simulink model "PMSM_Sensorless_ASMO_PLL"  (R2024b)
settings: Solver=FixedStepAuto  StartTime=0.0  StopTime=0.2  FixedStep=1e-6  RelTol=1e-3
model workspace (MAT data in the model file):
  B = 0
  Current_Filter_On = 0
  F = 10000
  J = 5.8e-05
  Ls = 0.0005125
  PLL_Ki = 800
  PLL_Kp = 1000
  Pn = 5
  Rs = 0.1445
  T_deadband = 0
  Ts = 5e-05
  Vdc = 60
  id_ki = 5
  id_kp = 2.5
  iq_ki = 5
  iq_kp = 2.5
  k = 150
  l_asmo = 2000
  psi_f = 0.0113
  speed_ki = 5
  speed_kp = 0.2
  w_c = 8000
undefined symbols (not defined in the file): sigbuilder_block
libraries: dspfdesign x3, slpidlib x3, simulink x2, spsDCVoltageSourceLib x1, spsOnDelayLib x1, spsGroundLib x1, dsparch4 x1, spsPermanentMagnetSynchronousMachineLib x1, spsThreePhaseVIMeasurementLib x1, spsTwoLevelConverterLib x1, spspowerguiLib x1
settings Model: Creator=A  LastModifiedBy=31904
settings OptimizationCC: ReuseModelBlockBuffer=off
settings ModelReferenceCC: EnableRefExpFcnMdlSchedulingChecks=on
settings RTWCC: GPUComputeCapability=3.5

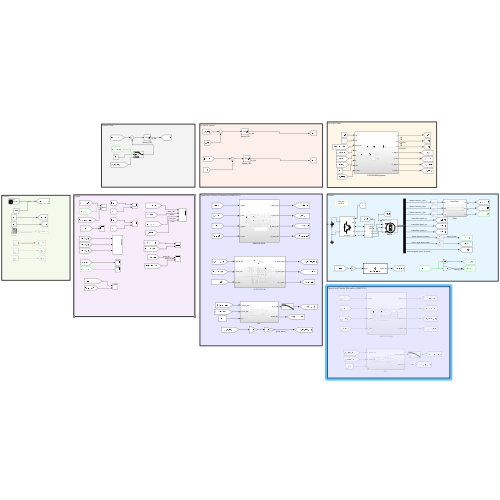
[thumbnail: Simulink's stored preview of the top-level diagram]
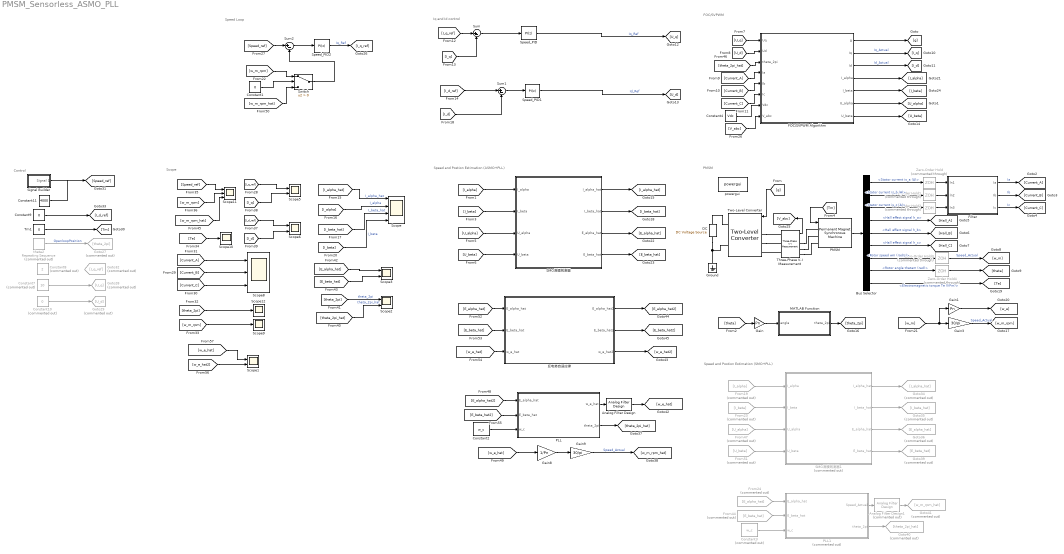
== system PMSM_Sensorless_ASMO_PLL ==
  note: Speed and Postion Estimation (ASMO+PLL)
  note: Iq and Id control
  note: FOC/SVPWM
  note: PMSM
  note: Speed Loop
  note: Control
  note: Scope
  note: Speed and Postion Estimation (SMO+PLL)
  Analog Filter Design : dspfdesign/Analog Filter Design  method=Butterworth  filttype=Lowpass  N=1  Wlo=8000  Whi=80  Rp=2  Rs=40
  Analog Filter Design1 : dspfdesign/Analog Filter Design  Commented=on  method=Butterworth  filttype=Lowpass  N=1  Wlo=8000  Whi=80  Rp=2  Rs=40
  Bus Selector : BusSelector  OutputSignals=Stator current is_a (A),Stator current is_b (A),Stator current is_c (A),Hall effect signal h_a,Hall effect signal h_b,Hall effect signal h_c,Rotor speed wm (rad/s),Rotor angle thetam (rad),Electromagnetic torque Te (N*m)
  Constant1 : Constant  Value=0
  Constant10 : Constant  Commented=on  Value=0
  Constant11 : Constant  Value=4000
  Constant2 : Constant  Value=w_c
  Constant3 : Constant  Commented=on  Value=w_c
  Constant4 : Constant  Value=Vdc
  Constant7 : Constant  Commented=on  Value=10
  Constant8 : Constant  Commented=on  Value=2
  Constant9 : Constant  Value=0
  DC : spsDCVoltageSourceLib/DC Voltage Source  Amplitude=Vdc  Measurements=None
  FOC/SVPWM Algorithm : Subsystem
  Filter : Subsystem  Variant=on
  From19 : From  Commented=on  GotoTag=I_alpha
  From23 : From  Commented=on  GotoTag=I_beta
  From24 : From  Commented=on  GotoTag=E_alpha_hat
  From44 : From  Commented=on  GotoTag=E_beta_hat
  From47 : From  Commented=on  GotoTag=U_alpha
  From51 : From  Commented=on  GotoTag=U_beta
  Gain : Gain  Gain=Pn
  Gain1 : Gain  Gain=Pn
  Gain3 : Gain  Gain=30/pi
  Gain8 : Gain  Gain=1/Pn
  Gain9 : Gain  Gain=30/pi
  Goto27 : Goto  Commented=on  GotoTag=theta_2pi
  Goto28 : Goto  Commented=on  GotoTag=U_q
  Goto29 : Goto  Commented=on  GotoTag=U_d
  Goto32 : Goto  Commented=on  GotoTag=I_q_ref
  Goto34 : Goto  Commented=on  GotoTag=I_alpha_hat
  Goto35 : Goto  Commented=on  GotoTag=I_beta_hat
  Goto36 : Goto  Commented=on  GotoTag=E_alpha_hat
  Goto39 : Goto  Commented=on  GotoTag=E_beta_hat
  Goto40 : Goto  Commented=on  GotoTag=theta_2pi_hat
  Goto41 : Goto  Commented=on  GotoTag=w_m_rpm_hat
  Ground : spsGroundLib/Ground  LConnTagsString=a
  MATLAB Function : MATLAB Function  TreatAsAtomicUnit=on
  PLL : Subsystem
  PLL1 : Subsystem  Commented=on
  PMSM : spsPermanentMagnetSynchronousMachineLib/Permanent Magnet Synchronous Machine  NbPhases=3  FluxDistribution=Sinusoidal  RotorType=Round  MechanicalLoad=Torque Tm  PresetModel=No  ShowDetailedParameters=on  MeasurementBus=off  Resistance=Rs  Inductance=8.5e-3  dqInductances=[8.5e-3,8.5e-3]  La=Ls  MachineConstant=Flux linkage established by magnets (V.s)  Flux=psi_f  VoltageCst=10.248  TorqueCst=0.08475  Flat=120  Mechanical=[J B Pn 0]  PolePairs=4  InitialConditions=[0,0, 0,0]  InitialConditions5ph=[0 0 0 0 0 0]  RefAngle=Aligned with phase A axis (original Park)  IterativeDiscreteModel=Trapezoidal non iterative  TsBlock=-1  TsPowergui=0
  SMO滑膜观测器 : Subsystem
  SMO滑膜观测器1 : Subsystem  Commented=on
  Scope : Scope  NumInputPorts=4
  Scope{1..3,5..6} (5 alike) : Scope  NumInputPorts=2
  Scope10 : Scope
  Scope11 : Scope  NumInputPorts=3
  Scope12 : Scope
  Scope8 : Scope  NumInputPorts=3
  Scope9 : Scope
  Signal Builder : Subsystem  Tag=STV Subsys  LoadFcn=sigbuilder_block('load');  StartFcn=sigbuilder_block('start');  StopFcn=sigbuilder_block('stop');  ClipboardFcn=sigbuilder_block('clipboard');  mask(Sigbuilder block){tuvar=[0:10]}
      mask help: Simulink:masks:SigbuilderBlock_MD
      mask init:
      | if ~strcmp(get_param(bdroot(gcbh),'SimulationStatus'),'stopped') tuvar = sigbuilder_block('maskInit'); end
      settings: CopyFcn=sigbuilder_block('copy');  DeleteFcn=sigbuilder_block('delete');  ModelCloseFcn=sigbuilder_block('modelClose');  PreSaveFcn=sigbuilder_block('preSave');  PauseFcn=sigbuilder_block('pause');  ContinueFcn=sigbuilder_block('continue');  NameChangeFcn=sigbuilder_block('namechange');  OpenFcn=sigbuilder_block('open',[458.1 40.8 550.2 399.9 ]);  CloseFcn=sigbuilder_block('close');
      mask Display: plot(0, 0, 100, 100,[2, 2, 32, 32, 2], [68, 8, 8, 68, 68],[32, 2], [38, 38], [32, 19, 2],[53, 60, 44], [32, 17, 17, 2],[16, 16, 31, 31]);txt = getActiveGroup(gcbh);text(2, 100, txt,'verticalAlignment', 'top');
  Speed_PID : slpidlib/PID Controller  Controller=PI  Form=Parallel  TimeDomain=Discrete-time  UseExternalTs=off  SampleTime=-1  IntegratorMethod=Forward Euler  FilterMethod=Forward Euler  ControllerParametersSource=internal  P=iq_kp  I=iq_ki  UseKiTs=off  D=0  UseExternalDerivativeSource=off  N=100  UseFilter=on  TunerSelectOption=Transfer Function Based (PID Tuner App)  InitialConditionSource=internal  InitialConditionForIntegrator=0  InitialConditionForFilter=0  DifferentiatorICPrevScaledInput=0  ExternalReset=none  TrackingMode=off  Kt=1  LimitOutput=on  SatLimitsSource=internal  UpperSaturationLimit=Vdc  LowerSaturationLimit=-Vdc  LinearizeAsGain=off  AntiWindupMode=back-calculation  Kb=0.9  LimitIntegrator=off  UpperIntegratorSaturationLimit=inf  LowerIntegratorSaturationLimit=-inf  POutMin=[]  POutMax=[]  IOutMin=[]  IOutMax=[]  DOutMin=[]  DOutMax=[]  NOutMin=[]  NOutMax=[]  SumOutMin=[]  SumOutMax=[]  SaturationOutMin=[]  SaturationOutMax=[]  PParamMin=[]  PParamMax=[]  IParamMin=[]  IParamMax=[]  DParamMin=[]  DParamMax=[]  NParamMin=[]  NParamMax=[]  KbParamMin=[]  KbParamMax=[]  KtParamMin=[]  KtParamMax=[]  KbOutMin=[]  KbOutMax=[]  KtOutMin=[]  KtOutMax=[]  IntegratorOutMin=[]  IntegratorOutMax=[]  FilterOutMin=[]  FilterOutMax=[]  SumI1OutMin=[]  SumI1OutMax=[]  SumI2OutMin=[]  SumI2OutMax=[]  SumI3OutMin=[]  SumI3OutMax=[]  SumI4OutMin=[]  SumI4OutMax=[]  SumDOutMin=[]  SumDOutMax=[]  DifferentiatorOutMin=[]  DifferentiatorOutMax=[]  FilterDiffOutCoefMin=[]  FilterDiffOutCoefMax=[]  ReciprocalOutMin=[]  ReciprocalOutMax=[]  SumDenOutMin=[]  SumDenOutMax=[]  SumNumOutMin=[]  SumNumOutMax=[]  DivideOutMin=[]  DivideOutMax=[]  UdiffTsProdOutMin=[]  UdiffTsProdOutMax=[]  NTsProdOutMin=[]  NTsProdOutMax=[]  UintegralTsProdOutMin=[]  UintegralTsProdOutMax=[]  UngainTsProdOutMin=[]  UngainTsProdOutMax=[]  ClampingZeroOutDataTypeStr=Inherit: Inherit via back propagation  ClampingZeroOutMin=[]  ClampingZeroOutMax=[]  FilterDenConstantOutDataTypeStr=Inherit: Inherit via back propagation  FilterDenConstantOutMin=[]  FilterDenConstantOutMax=[]  PCopyOutDataTypeStr=Inherit: Inherit via back propagation  PCopyOutMin=[]  PCopyOutMax=[]  NCopyOutDataTypeStr=Inherit: Inherit via back propagation  NCopyOutMin=[]  NCopyOutMax=[]  IntegratorContinuousStateAttributes=''  IntegratorStateMustResolveToSignalObject=off  IntegratorRTWStateStorageClass=Auto  FilterContinuousStateAttributes=''  FilterStateMustResolveToSignalObject=off  FilterRTWStateStorageClass=Auto  ParallelPVariant=InternalParameters  IdealPVariant=Disabled  IVariant=InternalParameters  DVariant=Disabled  IntegratorVariant=Discrete  SatVariant=Enabled  AWVariant=BackCalculation  PCopyVariant=Disabled  TRVariant=Disabled  FdbkBlocksVariant=Forward  IdealPFdbkVariant=Disabled  SatFdbkVariant=Disabled  DerivativeFilterVariant=Disabled  NVariant=Disabled  NCopyVariant=Disabled_SignalSpec  FilterICVariant=Disabled  IntegratorICVariant=InternalICs  ExternalResetVariant=Disabled  TRSumVariant=Passthrough  SumFdbkVariant=Disabled  SumVariant=Sum_PI  TsampFilterVariant=InternalTs  TsampNgainVariant=Passthrough  TsampIntegralVariant=Disabled_SignalSpec  ExternalSaturationOutDataTypeStr=Inherit: Same as second input  DerivativeSourceVariant=Disabled  PreIntVariant=InternalPreInt
  Speed_PID1 : slpidlib/PID Controller  Controller=PI  Form=Parallel  TimeDomain=Discrete-time  UseExternalTs=off  SampleTime=-1  IntegratorMethod=Forward Euler  FilterMethod=Forward Euler  ControllerParametersSource=internal  P=id_kp  I=id_ki  UseKiTs=off  D=0  UseExternalDerivativeSource=off  N=100  UseFilter=on  TunerSelectOption=Transfer Function Based (PID Tuner App)  InitialConditionSource=internal  InitialConditionForIntegrator=0  InitialConditionForFilter=0  DifferentiatorICPrevScaledInput=0  ExternalReset=none  TrackingMode=off  Kt=1  LimitOutput=on  SatLimitsSource=internal  UpperSaturationLimit=Vdc  LowerSaturationLimit=-Vdc  LinearizeAsGain=off  AntiWindupMode=back-calculation  Kb=0.8  LimitIntegrator=off  UpperIntegratorSaturationLimit=inf  LowerIntegratorSaturationLimit=-inf  POutMin=[]  POutMax=[]  IOutMin=[]  IOutMax=[]  DOutMin=[]  DOutMax=[]  NOutMin=[]  NOutMax=[]  SumOutMin=[]  SumOutMax=[]  SaturationOutMin=[]  SaturationOutMax=[]  PParamMin=[]  PParamMax=[]  IParamMin=[]  IParamMax=[]  DParamMin=[]  DParamMax=[]  NParamMin=[]  NParamMax=[]  KbParamMin=[]  KbParamMax=[]  KtParamMin=[]  KtParamMax=[]  KbOutMin=[]  KbOutMax=[]  KtOutMin=[]  KtOutMax=[]  IntegratorOutMin=[]  IntegratorOutMax=[]  FilterOutMin=[]  FilterOutMax=[]  SumI1OutMin=[]  SumI1OutMax=[]  SumI2OutMin=[]  SumI2OutMax=[]  SumI3OutMin=[]  SumI3OutMax=[]  SumI4OutMin=[]  SumI4OutMax=[]  SumDOutMin=[]  SumDOutMax=[]  DifferentiatorOutMin=[]  DifferentiatorOutMax=[]  FilterDiffOutCoefMin=[]  FilterDiffOutCoefMax=[]  ReciprocalOutMin=[]  ReciprocalOutMax=[]  SumDenOutMin=[]  SumDenOutMax=[]  SumNumOutMin=[]  SumNumOutMax=[]  DivideOutMin=[]  DivideOutMax=[]  UdiffTsProdOutMin=[]  UdiffTsProdOutMax=[]  NTsProdOutMin=[]  NTsProdOutMax=[]  UintegralTsProdOutMin=[]  UintegralTsProdOutMax=[]  UngainTsProdOutMin=[]  UngainTsProdOutMax=[]  ClampingZeroOutDataTypeStr=Inherit: Inherit via back propagation  ClampingZeroOutMin=[]  ClampingZeroOutMax=[]  FilterDenConstantOutDataTypeStr=Inherit: Inherit via back propagation  FilterDenConstantOutMin=[]  FilterDenConstantOutMax=[]  PCopyOutDataTypeStr=Inherit: Inherit via back propagation  PCopyOutMin=[]  PCopyOutMax=[]  NCopyOutDataTypeStr=Inherit: Inherit via back propagation  NCopyOutMin=[]  NCopyOutMax=[]  IntegratorContinuousStateAttributes=''  IntegratorStateMustResolveToSignalObject=off  IntegratorRTWStateStorageClass=Auto  FilterContinuousStateAttributes=''  FilterStateMustResolveToSignalObject=off  FilterRTWStateStorageClass=Auto  ParallelPVariant=InternalParameters  IdealPVariant=Disabled  IVariant=InternalParameters  DVariant=Disabled  IntegratorVariant=Discrete  SatVariant=Enabled  AWVariant=BackCalculation  PCopyVariant=Disabled  TRVariant=Disabled  FdbkBlocksVariant=Forward  IdealPFdbkVariant=Disabled  SatFdbkVariant=Disabled  DerivativeFilterVariant=Disabled  NVariant=Disabled  NCopyVariant=Disabled_SignalSpec  FilterICVariant=Disabled  IntegratorICVariant=InternalICs  ExternalResetVariant=Disabled  TRSumVariant=Passthrough  SumFdbkVariant=Disabled  SumVariant=Sum_PI  TsampFilterVariant=InternalTs  TsampNgainVariant=Passthrough  TsampIntegralVariant=Disabled_SignalSpec  ExternalSaturationOutDataTypeStr=Inherit: Same as second input  DerivativeSourceVariant=Disabled  PreIntVariant=InternalPreInt
  Speed_PID2 : slpidlib/PID Controller  Controller=PI  Form=Parallel  TimeDomain=Discrete-time  UseExternalTs=off  SampleTime=-1  IntegratorMethod=Forward Euler  FilterMethod=Forward Euler  ControllerParametersSource=internal  P=speed_kp  I=speed_ki  UseKiTs=off  D=0  UseExternalDerivativeSource=off  N=100  UseFilter=on  TunerSelectOption=Transfer Function Based (PID Tuner App)  InitialConditionSource=internal  InitialConditionForIntegrator=0  InitialConditionForFilter=0  DifferentiatorICPrevScaledInput=0  ExternalReset=none  TrackingMode=off  Kt=1  LimitOutput=on  SatLimitsSource=internal  UpperSaturationLimit=Vdc  LowerSaturationLimit=-Vdc  LinearizeAsGain=on  AntiWindupMode=back-calculation  Kb=10  LimitIntegrator=off  UpperIntegratorSaturationLimit=inf  LowerIntegratorSaturationLimit=-inf  POutMin=[]  POutMax=[]  IOutMin=[]  IOutMax=[]  DOutMin=[]  DOutMax=[]  NOutMin=[]  NOutMax=[]  SumOutMin=[]  SumOutMax=[]  SaturationOutMin=[]  SaturationOutMax=[]  PParamMin=[]  PParamMax=[]  IParamMin=[]  IParamMax=[]  DParamMin=[]  DParamMax=[]  NParamMin=[]  NParamMax=[]  KbParamMin=[]  KbParamMax=[]  KtParamMin=[]  KtParamMax=[]  KbOutMin=[]  KbOutMax=[]  KtOutMin=[]  KtOutMax=[]  IntegratorOutMin=[]  IntegratorOutMax=[]  FilterOutMin=[]  FilterOutMax=[]  SumI1OutMin=[]  SumI1OutMax=[]  SumI2OutMin=[]  SumI2OutMax=[]  SumI3OutMin=[]  SumI3OutMax=[]  SumI4OutMin=[]  SumI4OutMax=[]  SumDOutMin=[]  SumDOutMax=[]  DifferentiatorOutMin=[]  DifferentiatorOutMax=[]  FilterDiffOutCoefMin=[]  FilterDiffOutCoefMax=[]  ReciprocalOutMin=[]  ReciprocalOutMax=[]  SumDenOutMin=[]  SumDenOutMax=[]  SumNumOutMin=[]  SumNumOutMax=[]  DivideOutMin=[]  DivideOutMax=[]  UdiffTsProdOutMin=[]  UdiffTsProdOutMax=[]  NTsProdOutMin=[]  NTsProdOutMax=[]  UintegralTsProdOutMin=[]  UintegralTsProdOutMax=[]  UngainTsProdOutMin=[]  UngainTsProdOutMax=[]  ClampingZeroOutDataTypeStr=Inherit: Inherit via back propagation  ClampingZeroOutMin=[]  ClampingZeroOutMax=[]  FilterDenConstantOutDataTypeStr=Inherit: Inherit via back propagation  FilterDenConstantOutMin=[]  FilterDenConstantOutMax=[]  PCopyOutDataTypeStr=Inherit: Inherit via back propagation  PCopyOutMin=[]  PCopyOutMax=[]  NCopyOutDataTypeStr=Inherit: Inherit via back propagation  NCopyOutMin=[]  NCopyOutMax=[]  IntegratorContinuousStateAttributes=''  IntegratorStateMustResolveToSignalObject=off  IntegratorRTWStateStorageClass=Auto  FilterContinuousStateAttributes=''  FilterStateMustResolveToSignalObject=off  FilterRTWStateStorageClass=Auto  ParallelPVariant=InternalParameters  IdealPVariant=Disabled  IVariant=InternalParameters  DVariant=Disabled  IntegratorVariant=Discrete  SatVariant=Enabled  AWVariant=BackCalculation  PCopyVariant=Disabled  TRVariant=Disabled  FdbkBlocksVariant=Forward  IdealPFdbkVariant=Disabled  SatFdbkVariant=Disabled  DerivativeFilterVariant=Disabled  NVariant=Disabled  NCopyVariant=Disabled_SignalSpec  FilterICVariant=Disabled  IntegratorICVariant=InternalICs  ExternalResetVariant=Disabled  TRSumVariant=Passthrough  SumFdbkVariant=Disabled  SumVariant=Sum_PI  TsampFilterVariant=InternalTs  TsampNgainVariant=Passthrough  TsampIntegralVariant=Disabled_SignalSpec  ExternalSaturationOutDataTypeStr=Inherit: Same as second input  DerivativeSourceVariant=Disabled  PreIntVariant=InternalPreInt
  Sum : Sum  Inputs=|+-
  Sum1 : Sum  Inputs=|+-
  Sum2 : Sum  Inputs=|+-
  Switch : Switch  Criteria=u2 > Threshold  SaturateOnIntegerOverflow=off  InputSameDT=off
  Three-Phase V-I Measurement : spsThreePhaseVIMeasurementLib/Three-Phase V-I Measurement  VoltageMeasurement=phase-to-ground  SetLabelV=off  LabelV=Vabc  Vpu=off  VpuLL=off  CurrentMeasurement=yes  SetLabelI=off  LabelI=Iabc  Ipu=off  Pbase=100e6  Vbase=500e3  OutputType=Complex  PhasorSimulation=off  PSBequivalent=0
  Tm1 : Constant  Value=0
  Two-Level Converter : spsTwoLevelConverterLib/Two-Level Converter  ModelType=Switching devices  Ron=1e-3  Rs=1e6  Cs=inf  Vforward=[0,0]  Ron_Diode=1e-3  Rs_Diode=1e6  Cs_Diode=inf  Vf_Diode=1e-3  Rs_CurrentSource=inf  Ron_ACsource=1e-3
  Zero-Order Hold{,1..4} (5 alike) : ZeroOrderHold  Commented=through  SampleTime=1/F
  powergui : spspowerguiLib/powergui  Priority=1  SimulationMode=Discrete  SampleTime=1e-6  frequency=60  Iterations=50  frequencyindice=0  Pbase=100e6  ErrMax=1e-4  UnitsV=kV  UnitsW=MW  buscounter=0  FunctionMessages=off  echomessages=off  EnableUseOfTLC=off  CurrentSourceSwitches=off  DisableSnubberDevices=off  DisableRonSwitches=off  DisableVfSwitches=off  DisplayEquations=off  AutomaticDiscreteSolvers=off  SolverType=Tustin/Backward Euler (TBE)  Interpol=off  ExternalGateDelay=off  methode=off  Ts=100  x0status=blocks  SPID=on  SwTol=0  HookPort=off  NonlinearTolerance=1e-4  nMaxIteration=100  ContinueOnMaxIteration=off  RestoreLinks=warning  ResistiveCurrentMeasurement=off  Frange=[0:2:500]  Ylog=off  Xlog=on  ShowGrid=off  save=off  variable=ZData  structure=0  ZoomFFT=off  StartTime=0.0  cycles=1  DisplayStyle=1  fundamental=60  FreqAxis=off  MaxFrequency=1000  frequencyindicesteady=1  RmsSteady=1  display=off
  theta2 : simulink/Sources/Repeating Sequence  Commented=on  rep_seq_t=[0 0.1]  rep_seq_y=[0 2*pi]
  反电势自适应律 : Subsystem
  wires:
  Constant4/1 -> FOC/SVPWM Algorithm/7(Vdc)
  FOC/SVPWM Algorithm/3(Id) -> [I_d]  "Id_Actual"
  [U_d] -> FOC/SVPWM Algorithm/2(Ud)
  [U_q] -> FOC/SVPWM Algorithm/1(Uq)
  [Current_A] -> FOC/SVPWM Algorithm/4(Ia)
  [Current_C] -> FOC/SVPWM Algorithm/6(Ic)
  FOC/SVPWM Algorithm/2(Iq) -> [I_q]  "Iq_Actual"
  [Current_B] -> FOC/SVPWM Algorithm/5(Ib)
  Zero-Order Hold4/1 -> [theta]
  Bus Selector/1 -> Zero-Order Hold/1  "<Stator current is_a (A)>"
  Zero-Order Hold/1 -> Filter/1(ln1)
  Zero-Order Hold1/1 -> Filter/2(ln2)
  Bus Selector/4 -> [Hall_A]  "<Hall effect signal h_a>"
  [theta] -> Gain/1
  Bus Selector/2 -> Zero-Order Hold1/1  "<Stator current is_b (A)>"
  [g] -> Two-Level Converter/1
  Bus Selector/3 -> Zero-Order Hold2/1  "<Stator current is_c (A)>"
  [Tm] -> PMSM/1
  Zero-Order Hold3/1 -> [w_m]  "Speed_Actual"
  Bus Selector/8 -> Zero-Order Hold4/1  "<Rotor angle thetam (rad)>"
  MATLAB Function/1(theta_2pi) -> [theta_2pi]
  Bus Selector/7 -> Zero-Order Hold3/1  "<Rotor speed wm (rad/s)>"
  PMSM/1 -> Bus Selector/1
  Bus Selector/5 -> [Hall_B]  "<Hall effect signal h_b>"
  Zero-Order Hold2/1 -> Filter/3(ln3)
  Bus Selector/6 -> [Hall_C]  "<Hall effect signal h_c>"
  [I_q_ref] -> Sum/1
  [I_q] -> Sum/2
  Sum/1 -> Speed_PID/1
  Filter/1(Ia) -> [Current_A]  "Ia"
  Filter/2(Ib) -> [Current_B]  "Ib"
  Filter/3(Ic) -> [Current_C]  "Ic"
  FOC/SVPWM Algorithm/1(g) -> [g]
  Sum1/1 -> Speed_PID1/1
  [I_d] -> Sum1/2
  [I_d_ref] -> Sum1/1
  [w_m] -> Gain1/1, Gain3/1
  Gain3/1 -> [w_m_rpm]  "Speed_Actual"
  Gain/1 -> MATLAB Function/1(angle)
  Bus Selector/9 -> [Te]  "<Electromagnetic torque Te (N*m)>"
  FOC/SVPWM Algorithm/4(I_alpha) -> [I_alpha]
  FOC/SVPWM Algorithm/5(I_beta) -> [I_beta]
  Three-Phase V-I Measurement/1 -> [V_abc]
  [V_abc] -> FOC/SVPWM Algorithm/8(V_abc)
  Speed_PID2/1 -> [I_q_ref]  "Iq_Ref"
  [Speed_ref] -> Sum2/1
  Sum2/1 -> Speed_PID2/1
  Constant11/1 -> [Speed_ref]
  [w_m_rpm] -> Scope11/2
  [Te] -> Scope10/1
  Signal Builder/1(Signal 1) -> ?
  [Speed_ref] -> Scope11/1
  [I_q_ref] -> Scope5/1
  theta2/1 -> Goto27/1  "OpenloopPosition"
  [theta_2pi] -> Scope12/1
  [I_d_ref] -> Scope6/1
  Tm1/1 -> [Tm]
  [w_m_rpm] -> Scope9/1
  [Current_C] -> Scope8/3
  [Current_B] -> Scope8/2
  [Current_A] -> Scope8/1
  [I_d] -> Scope6/2
  ? -> Goto32/1
  Constant7/1 -> Goto28/1
  Constant10/1 -> Goto29/1
  [I_q] -> Scope5/2
  Constant9/1 -> [I_d_ref]
  FOC/SVPWM Algorithm/6(U_alpha) -> [U_alpha]
  FOC/SVPWM Algorithm/7(U_beta) -> [U_beta]
  [I_alpha_hat] -> Scope/1  "I_alpha_hat"
  [I_alpha] -> Scope/2  "I_alpha"
  [I_beta_hat] -> Scope/3  "I_beta_hat"
  [I_beta] -> Scope/4  "I_beta"
  [I_alpha] -> SMO滑膜观测器/1(I_alpha)
  [I_beta] -> SMO滑膜观测器/2(I_beta)
  [U_alpha] -> SMO滑膜观测器/3(U_alpha)
  [U_beta] -> SMO滑膜观测器/4(U_beta)
  SMO滑膜观测器/1(I_alpha_hat) -> [I_alpha_hat]
  SMO滑膜观测器/2(I_beta_hat) -> [I_beta_hat]
  SMO滑膜观测器/3(E_alpha_hat) -> [E_alpha_hat]
  SMO滑膜观测器/4(E_beta_hat) -> [E_beta_hat]
  [theta_2pi] -> Scope2/1  "theta_2pi"
  [theta_2pi_hat] -> Scope2/2  "theta_2pi_hat"
  [E_alpha_hat] -> Scope3/1
  [E_beta_hat] -> Scope3/2
  Gain1/1 -> [w_e]
  [theta_2pi_hat] -> FOC/SVPWM Algorithm/3(theta_2pi)
  [w_m_rpm_hat] -> Scope11/3
  [w_m_rpm_hat] -> Switch/3
  [E_alpha_hat2] -> PLL/1(E_alpha_hat)
  [E_beta_hat2] -> PLL/2(E_beta_hat)
  PLL/1(w_e_hat) -> Analog Filter Design/1
  PLL/2(theta_2pi) -> [theta_2pi_hat]
  Analog Filter Design/1 -> [w_e_hat]
  [w_m_rpm] -> Switch/1
  Constant1/1 -> Switch/2
  Switch/1 -> Sum2/2
  Constant2/1 -> PLL/3(w_c)
  SMO滑膜观测器1/3(E_alpha_hat) -> Goto36/1
  SMO滑膜观测器1/1(I_alpha_hat) -> Goto34/1
  From47/1 -> SMO滑膜观测器1/3(U_alpha)
  From19/1 -> SMO滑膜观测器1/1(I_alpha)
  SMO滑膜观测器1/2(I_beta_hat) -> Goto35/1
  PLL1/1(Speed_Actual) -> Analog Filter Design1/1
  Constant3/1 -> PLL1/3(w_c)
  From24/1 -> PLL1/1(E_alpha_hat)
  SMO滑膜观测器1/4(E_beta_hat) -> Goto39/1
  PLL1/2(theta_2pi) -> Goto40/1
  From44/1 -> PLL1/2(E_beta_hat)
  Analog Filter Design1/1 -> Goto41/1
  From51/1 -> SMO滑膜观测器1/4(U_beta)
  From23/1 -> SMO滑膜观测器1/2(I_beta)
  Gain8/1 -> Gain9/1
  Gain9/1 -> [w_m_rpm_hat]  "Speed_Actual"
  [w_e_hat] -> Gain8/1
  [E_alpha_hat] -> 反电势自适应律/1(E_alpha_hat)
  [E_beta_hat] -> 反电势自适应律/2(E_beta_hat)
  [w_e_hat] -> 反电势自适应律/3(w_e_hat)
  反电势自适应律/1(E_alpha_hat2) -> [E_alpha_hat2]
  反电势自适应律/2(E_beta_hat2) -> [E_beta_hat2]
  反电势自适应律/3(w_e_hat2) -> [w_e_hat2]
  [w_e_hat2] -> Scope1/2
  [w_e_hat] -> Scope1/1
  Speed_PID1/1 -> [U_d]  "Id_Ref"
  Speed_PID/1 -> [U_q]  "Iq_Ref"
  connections:
  DC/LConn1 -- Two-Level Converter/RConn2 -- Ground/LConn1
  DC/RConn1 -- Two-Level Converter/RConn1
  Three-Phase V-I Measurement/LConn3 -- Two-Level Converter/LConn3
  Two-Level Converter/LConn1 -- Three-Phase V-I Measurement/LConn1
  Two-Level Converter/LConn2 -- Three-Phase V-I Measurement/LConn2
  Three-Phase V-I Measurement/RConn1 -- PMSM/LConn1
  Three-Phase V-I Measurement/RConn2 -- PMSM/LConn2
  Three-Phase V-I Measurement/RConn3 -- PMSM/LConn3

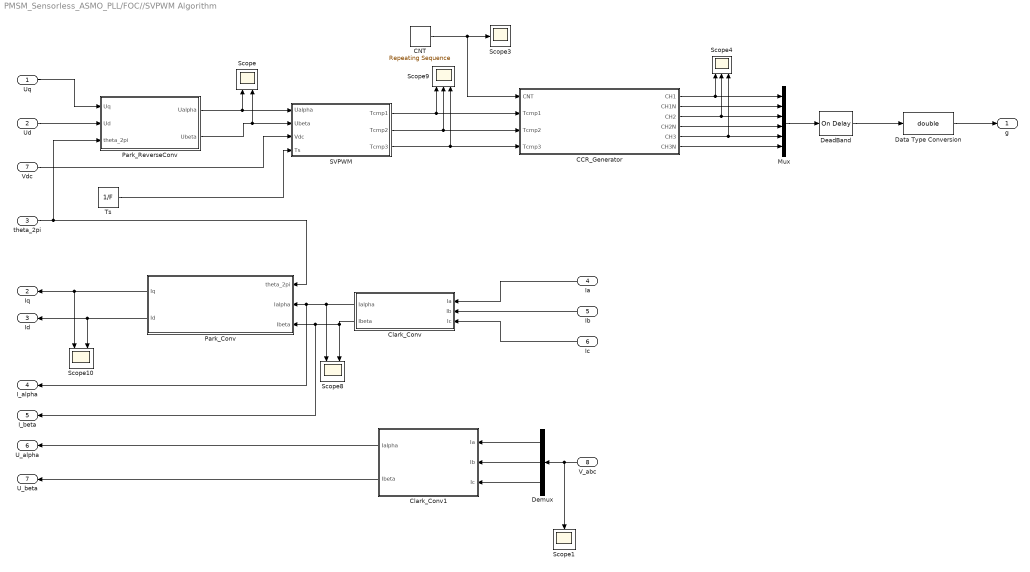
== system PMSM_Sensorless_ASMO_PLL/FOC//SVPWM Algorithm ==
  Uq : Inport
  Ud : Inport  Port=2
  theta_2pi : Inport  Port=3
  Ia : Inport  Port=4
  Ib : Inport  Port=5
  Ic : Inport  Port=6
  Vdc : Inport  Port=7
  V_abc : Inport  Port=8
  CCR_Generator : MATLAB Function  TreatAsAtomicUnit=on
  CNT : simulink/Sources/Repeating Sequence  rep_seq_t=[0 1/(2*F) 1/F]  rep_seq_y=[0 1/(2*F) 0]
  Clark_Conv : Subsystem
  Clark_Conv1 : Subsystem
  Data Type Conversion : DataTypeConversion  OutDataTypeStr=double  SaturateOnIntegerOverflow=off  RndMeth=Floor
  DeadBand : spsOnDelayLib/On Delay  DelayType=On delay  delay=T_deadband  ic=0  Ts=0
  Demux : Demux  Outputs=3
  Mux : Mux  Inputs=6
  Park_Conv : Subsystem
  Park_ReverseConv : Subsystem
  SVPWM : Subsystem
  Scope : Scope  NumInputPorts=2
  Scope1 : Scope
  Scope10 : Scope  NumInputPorts=2
  Scope3 : Scope
  Scope4 : Scope  NumInputPorts=3
  Scope8 : Scope  NumInputPorts=2
  Scope9 : Scope  NumInputPorts=3
  Ts : Constant  Value=1/F
  g : Outport
  Iq : Outport  Port=2
  Id : Outport  Port=3
  I_alpha : Outport  Port=4
  I_beta : Outport  Port=5
  U_alpha : Outport  Port=6
  U_beta : Outport  Port=7
  wires:
  Uq/1 -> Park_ReverseConv/1(Uq)
  SVPWM/3(Tcmp3) -> CCR_Generator/4(Tcmp3), Scope9/3
  Clark_Conv/1(Ialpha) -> I_alpha/1, Park_Conv/2(Ialpha), Scope8/1
  CCR_Generator/3(CH2) -> Mux/3, Scope4/2
  SVPWM/2(Tcmp2) -> CCR_Generator/3(Tcmp2), Scope9/2
  CCR_Generator/2(CH1N) -> Mux/2
  theta_2pi/1 -> Park_Conv/1(theta_2pi), Park_ReverseConv/3(theta_2pi)
  CCR_Generator/5(CH3) -> Mux/5, Scope4/3
  SVPWM/1(Tcmp1) -> CCR_Generator/2(Tcmp1), Scope9/1
  Clark_Conv/2(Ibeta) -> I_beta/1, Park_Conv/3(Ibeta), Scope8/2
  CCR_Generator/4(CH2N) -> Mux/4
  Park_ReverseConv/1(Ualpha) -> SVPWM/1(Ualpha), Scope/1
  CCR_Generator/6(CH3N) -> Mux/6
  Mux/1 -> DeadBand/1
  Park_ReverseConv/2(Ubeta) -> Scope/2, SVPWM/2(Ubeta)
  CNT/1 -> Scope3/1, CCR_Generator/1(CNT)
  Park_Conv/2(Id) -> Scope10/2, Id/1
  CCR_Generator/1(CH1) -> Mux/1, Scope4/1
  Ud/1 -> Park_ReverseConv/2(Ud)
  Park_Conv/1(Iq) -> Scope10/1, Iq/1
  Data Type Conversion/1 -> g/1
  Vdc/1 -> SVPWM/3(Vdc)
  Ic/1 -> Clark_Conv/3(Ic)
  Ib/1 -> Clark_Conv/2(Ib)
  Ia/1 -> Clark_Conv/1(Ia)
  Ts/1 -> SVPWM/4(Ts)
  DeadBand/1 -> Data Type Conversion/1
  V_abc/1 -> Scope1/1, Demux/1
  Demux/1 -> Clark_Conv1/1(Ia)
  Demux/2 -> Clark_Conv1/2(Ib)
  Demux/3 -> Clark_Conv1/3(Ic)
  Clark_Conv1/1(Ialpha) -> U_alpha/1
  Clark_Conv1/2(Ibeta) -> U_beta/1

== system PMSM_Sensorless_ASMO_PLL/Filter ==
  note: 1) Add Subsystem or Model blocks as valid variant choices.
      | 2) You cannot connect blocks at this level. At simulation, connectivity is automatically
      | determined, based on the active variant and port name matching.
  ln1 : Inport
  ln2 : Inport  Port=2
  ln3 : Inport  Port=3
  LowpassFilter : Subsystem  VariantControl=Current_Filter_On==1
  NoneFilter : Subsystem  VariantControl=Current_Filter_On==0
  Ia : Outport
  Ib : Outport  Port=2
  Ic : Outport  Port=3

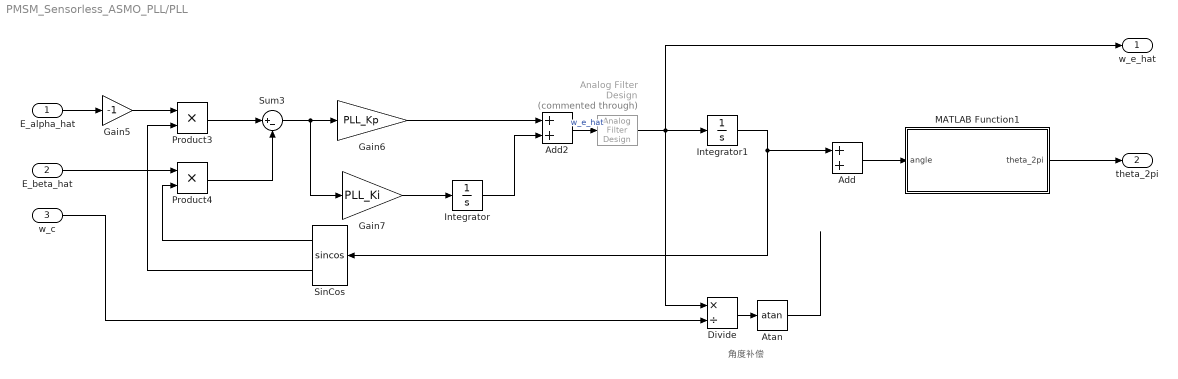
== system PMSM_Sensorless_ASMO_PLL/PLL ==
  note: 角度补偿
  E_alpha_hat : Inport
  E_beta_hat : Inport  Port=2
  w_c : Inport  Port=3
  Add : Sum
  Add2 : Sum
  Analog Filter Design : dspfdesign/Analog Filter Design  Commented=through  method=Butterworth  filttype=Lowpass  N=1  Wlo=1000  Whi=80  Rp=2  Rs=40
  Atan : Trigonometry  Operator=atan
  Divide : Product  Inputs=*/
  Gain5 : Gain  Gain=-1
  Gain6 : Gain  Gain=PLL_Kp
  Gain7 : Gain  Gain=PLL_Ki
  Integrator : Integrator
  Integrator1 : Integrator
  MATLAB Function1 : MATLAB Function  TreatAsAtomicUnit=on
  Product3 : Product
  Product4 : Product
  SinCos : Trigonometry  Operator=sincos
  Sum3 : Sum  Inputs=|+-
  w_e_hat : Outport
  theta_2pi : Outport  Port=2
  wires:
  Gain5/1 -> Product3/1
  Product4/1 -> Sum3/2
  Gain6/1 -> Add2/1
  Gain7/1 -> Integrator/1
  Sum3/1 -> Gain7/1, Gain6/1
  Product3/1 -> Sum3/1
  SinCos/2 -> Product3/2
  Add2/1 -> Analog Filter Design/1  "w_e_hat"
  Integrator1/1 -> Add/1, SinCos/1
  Integrator/1 -> Add2/2
  SinCos/1 -> Product4/2
  E_alpha_hat/1 -> Gain5/1
  E_beta_hat/1 -> Product4/1
  MATLAB Function1/1(theta_2pi) -> theta_2pi/1
  w_c/1 -> Divide/2
  Divide/1 -> Atan/1
  Add/1 -> MATLAB Function1/1(angle)
  Atan/1 -> ?
  Analog Filter Design/1 -> w_e_hat/1, Divide/1, Integrator1/1

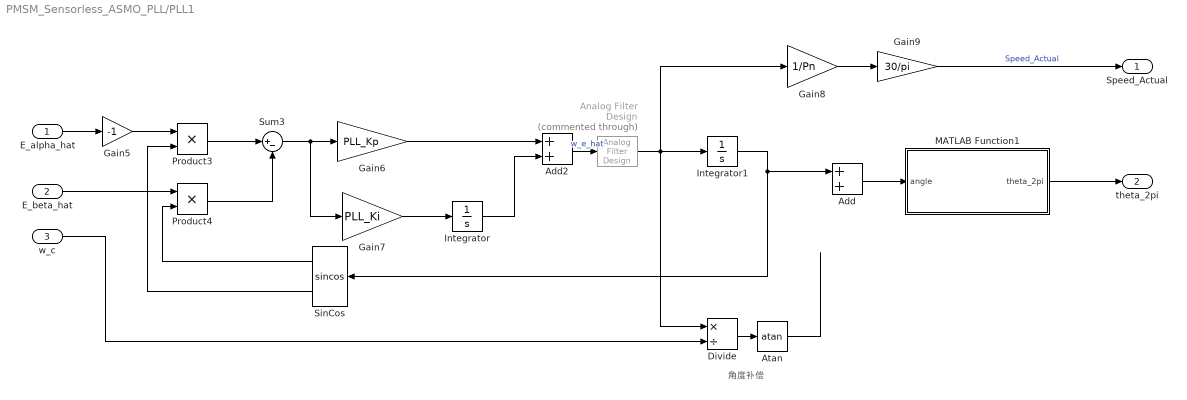
== system PMSM_Sensorless_ASMO_PLL/PLL1 ==
  note: 角度补偿
  E_alpha_hat : Inport
  E_beta_hat : Inport  Port=2
  w_c : Inport  Port=3
  Add : Sum
  Add2 : Sum
  Analog Filter Design : dsparch4/Analog Filter Design  Commented=through  method=Butterworth  filttype=Lowpass  N=1  Wlo=1000  Whi=80  Rp=2  Rs=40
  Atan : Trigonometry  Operator=atan
  Divide : Product  Inputs=*/
  Gain5 : Gain  Gain=-1
  Gain6 : Gain  Gain=PLL_Kp
  Gain7 : Gain  Gain=PLL_Ki
  Gain8 : Gain  Gain=1/Pn
  Gain9 : Gain  Gain=30/pi
  Integrator : Integrator
  Integrator1 : Integrator
  MATLAB Function1 : MATLAB Function  TreatAsAtomicUnit=on
  Product3 : Product
  Product4 : Product
  SinCos : Trigonometry  Operator=sincos
  Sum3 : Sum  Inputs=|+-
  Speed_Actual : Outport
  theta_2pi : Outport  Port=2
  wires:
  Gain5/1 -> Product3/1
  Gain8/1 -> Gain9/1
  Product4/1 -> Sum3/2
  Gain6/1 -> Add2/1
  Gain7/1 -> Integrator/1
  Sum3/1 -> Gain7/1, Gain6/1
  Product3/1 -> Sum3/1
  SinCos/2 -> Product3/2
  Add2/1 -> Analog Filter Design/1  "w_e_hat"
  Integrator1/1 -> Add/1, SinCos/1
  Integrator/1 -> Add2/2
  SinCos/1 -> Product4/2
  E_alpha_hat/1 -> Gain5/1
  E_beta_hat/1 -> Product4/1
  MATLAB Function1/1(theta_2pi) -> theta_2pi/1
  Gain9/1 -> Speed_Actual/1  "Speed_Actual"
  w_c/1 -> Divide/2
  Divide/1 -> Atan/1
  Add/1 -> MATLAB Function1/1(angle)
  Atan/1 -> ?
  Analog Filter Design/1 -> Gain8/1, Divide/1, Integrator1/1

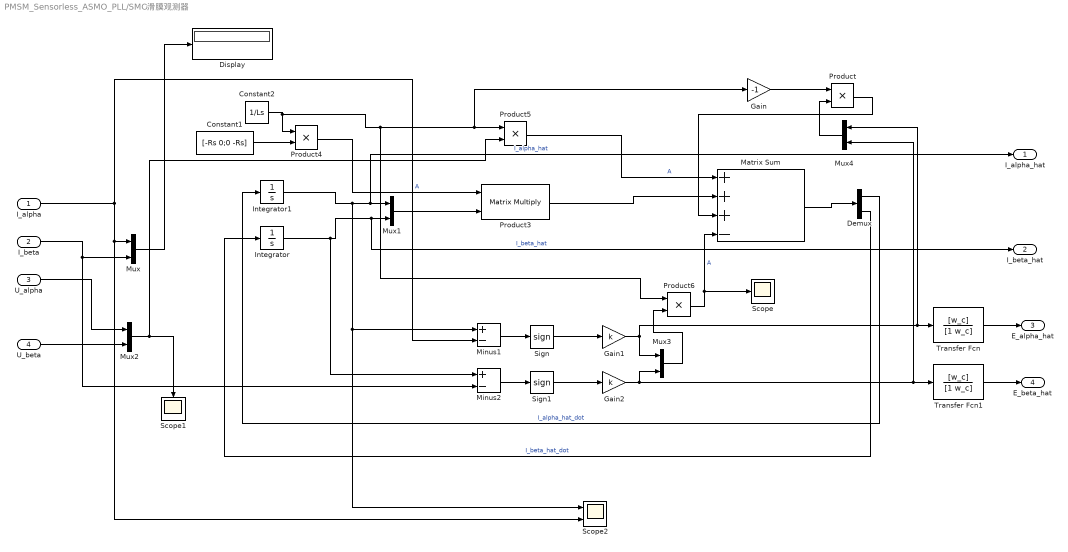
== system PMSM_Sensorless_ASMO_PLL/SMO滑膜观测器 ==
  I_alpha : Inport
  I_beta : Inport  Port=2
  U_alpha : Inport  Port=3
  U_beta : Inport  Port=4
  Constant1 : Constant  Value=[-Rs 0;0 -Rs]
  Constant2 : Constant  Value=1/Ls
  Demux : Demux  Outputs=2
  Display : Display
  Gain : Gain  Gain=-1
  Gain1 : Gain  Gain=k
  Gain2 : Gain  Gain=k
  Integrator : Integrator
  Integrator1 : Integrator
  Matrix Sum : Sum  Inputs=+++-
  Minus1 : Sum  Inputs=+-
  Minus2 : Sum  Inputs=+-
  Mux{,1..4} (5 alike) : Mux  Inputs=2
  Product{,4..6} (4 alike) : Product
  Product3 : Product  Multiplication=Matrix(*)
  Scope : Scope
  Scope1 : Scope
  Scope2 : Scope  NumInputPorts=2
  Sign : Signum
  Sign1 : Signum
  Transfer Fcn : TransferFcn  Numerator=[w_c]  Denominator=[1 w_c]
  Transfer Fcn1 : TransferFcn  Numerator=[w_c]  Denominator=[1 w_c]
  I_alpha_hat : Outport
  I_beta_hat : Outport  Port=2
  E_alpha_hat : Outport  Port=3
  E_beta_hat : Outport  Port=4
  wires:
  Mux/1 -> Display/1
  I_beta/1 -> Minus2/2, Mux/2
  Mux1/1 -> Product3/2
  I_alpha/1 -> Scope2/2, Mux/1, Minus1/2
  Constant2/1 -> Product6/1, Gain/1, Product5/1, Product4/1
  Mux2/1 -> Scope1/1, Product5/2
  Integrator1/1 -> Scope2/1, Minus1/1, I_alpha_hat/1, Mux1/1  "I_alpha_hat"
  Product6/1 -> Matrix Sum/4, Scope/1  "A"
  Minus2/1 -> Sign1/1
  Matrix Sum/1 -> Demux/1
  Integrator/1 -> Minus2/1, I_beta_hat/1, Mux1/2  "I_beta_hat"
  Constant1/1 -> Product4/2
  Sign1/1 -> Gain2/1
  Mux3/1 -> Product6/2
  Minus1/1 -> Sign/1
  Product3/1 -> Matrix Sum/2
  Product4/1 -> Product3/1  "A"
  Demux/2 -> Integrator/1  "I_beta_hat_dot"
  U_alpha/1 -> Mux2/1
  Demux/1 -> Integrator1/1  "I_alpha_hat_dot"
  Sign/1 -> Gain1/1
  Product5/1 -> Matrix Sum/1  "A"
  U_beta/1 -> Mux2/2
  Gain1/1 -> Mux4/1, Transfer Fcn/1, Mux3/1
  Gain2/1 -> Mux4/2, Transfer Fcn1/1, Mux3/2
  Transfer Fcn/1 -> E_alpha_hat/1
  Transfer Fcn1/1 -> E_beta_hat/1
  Gain/1 -> Product/1
  Mux4/1 -> Product/2
  Product/1 -> Matrix Sum/3

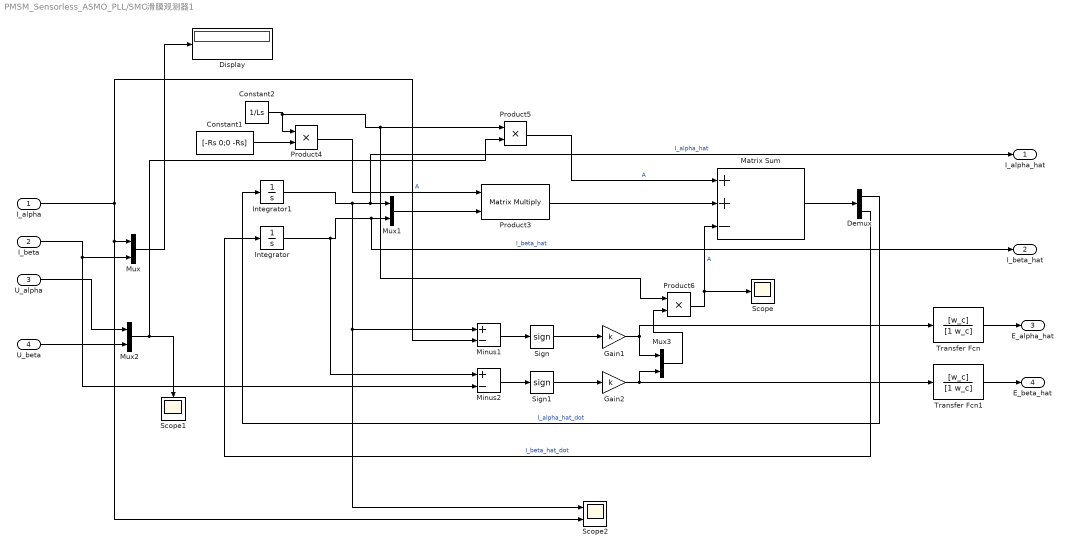
== system PMSM_Sensorless_ASMO_PLL/SMO滑膜观测器1 ==
  I_alpha : Inport
  I_beta : Inport  Port=2
  U_alpha : Inport  Port=3
  U_beta : Inport  Port=4
  Constant1 : Constant  Value=[-Rs 0;0 -Rs]
  Constant2 : Constant  Value=1/Ls
  Demux : Demux  Outputs=2
  Display : Display
  Gain1 : Gain  Gain=k
  Gain2 : Gain  Gain=k
  Integrator : Integrator
  Integrator1 : Integrator
  Matrix Sum : Sum  Inputs=++-
  Minus1 : Sum  Inputs=+-
  Minus2 : Sum  Inputs=+-
  Mux{,1..3} (4 alike) : Mux  Inputs=2
  Product3 : Product  Multiplication=Matrix(*)
  Product4 : Product
  Product5 : Product
  Product6 : Product
  Scope : Scope
  Scope1 : Scope
  Scope2 : Scope  NumInputPorts=2
  Sign : Signum
  Sign1 : Signum
  Transfer Fcn : TransferFcn  Numerator=[w_c]  Denominator=[1 w_c]
  Transfer Fcn1 : TransferFcn  Numerator=[w_c]  Denominator=[1 w_c]
  I_alpha_hat : Outport
  I_beta_hat : Outport  Port=2
  E_alpha_hat : Outport  Port=3
  E_beta_hat : Outport  Port=4
  wires:
  Mux/1 -> Display/1
  I_beta/1 -> Minus2/2, Mux/2
  Mux1/1 -> Product3/2
  I_alpha/1 -> Scope2/2, Mux/1, Minus1/2
  Constant2/1 -> Product6/1, Product5/1, Product4/1
  Mux2/1 -> Scope1/1, Product5/2
  Integrator1/1 -> Scope2/1, Minus1/1, I_alpha_hat/1, Mux1/1  "I_alpha_hat"
  Product6/1 -> Scope/1, Matrix Sum/3  "A"
  Minus2/1 -> Sign1/1
  Matrix Sum/1 -> Demux/1
  Integrator/1 -> Minus2/1, I_beta_hat/1, Mux1/2  "I_beta_hat"
  Constant1/1 -> Product4/2
  Sign1/1 -> Gain2/1
  Mux3/1 -> Product6/2
  Minus1/1 -> Sign/1
  Product3/1 -> Matrix Sum/2
  Product4/1 -> Product3/1  "A"
  Demux/2 -> Integrator/1  "I_beta_hat_dot"
  U_alpha/1 -> Mux2/1
  Demux/1 -> Integrator1/1  "I_alpha_hat_dot"
  Sign/1 -> Gain1/1
  Product5/1 -> Matrix Sum/1  "A"
  U_beta/1 -> Mux2/2
  Gain1/1 -> Transfer Fcn/1, Mux3/1
  Gain2/1 -> Transfer Fcn1/1, Mux3/2
  Transfer Fcn/1 -> E_alpha_hat/1
  Transfer Fcn1/1 -> E_beta_hat/1

== system PMSM_Sensorless_ASMO_PLL/Signal Builder ==
  Demux : Demux  Tag=STV Demux  Outputs=1
      settings: DisplayOption=none
  FromWs : FromWorkspace  Tag=STV FromWs  VariableName=tuvar
      SigBuilderData=|
      | common.afterFinalStr = 'Extrapolate'
      | common.sampleTime = 0
      | dataSet.timeRange = [0 1]
      | dataSet.name = 'Group 1'
      | sbobj.Groups.Name = 'Group 1'
      | sbobj.Groups.Signals.Name = 'Signal 1'
      | sbobj.Groups.Signals.XData = [0 0.2 0.2 0.3 0.3 0.5 0.5 0.6 0.6 0.8 0.8 0.9 0.9 1]
      | sbobj.Groups.Signals.YData = [1000 1000 3000 3000 5000 5000 4000 4000 2000 2000 1000 1000 0 0]
      | sbobj.Groups.TimeRange = [0 1]
  Signal 1 : Outport  Tag=STV Outport
  wires:
  Demux/1 -> Signal 1/1
  FromWs/1 -> Demux/1

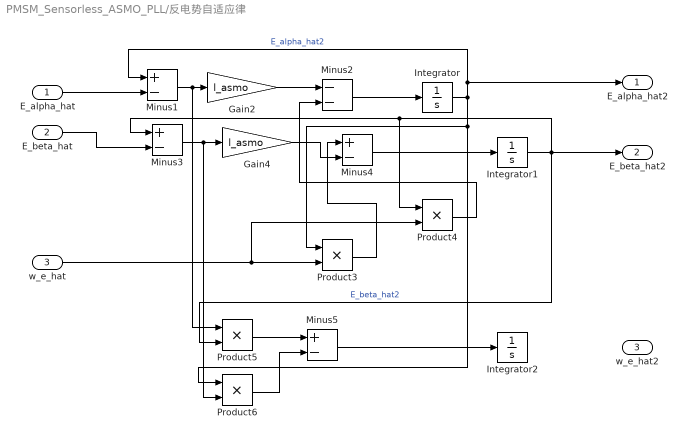
== system PMSM_Sensorless_ASMO_PLL/反电势自适应律 ==
  E_alpha_hat : Inport
  E_beta_hat : Inport  Port=2
  w_e_hat : Inport  Port=3
  Gain2 : Gain  Gain=l_asmo
  Gain4 : Gain  Gain=l_asmo
  Integrator : Integrator
  Integrator1 : Integrator
  Integrator2 : Integrator
  Minus{1,3..5} (4 alike) : Sum  Inputs=+-
  Minus2 : Sum  Inputs=--
  Product{3..6} (4 alike) : Product
  E_alpha_hat2 : Outport
  E_beta_hat2 : Outport  Port=2
  w_e_hat2 : Outport  Port=3
  wires:
  Minus5/1 -> Integrator2/1
  Gain4/1 -> Minus4/2
  Integrator/1 -> E_alpha_hat2/1, Minus1/1, Product6/1, Product3/1  "E_alpha_hat2"
  w_e_hat/1 -> Product4/2, Product3/2
  Integrator1/1 -> E_beta_hat2/1, Product5/2, Minus3/1, Product4/1  "E_beta_hat2"
  E_alpha_hat/1 -> Minus1/2
  Product4/1 -> Minus2/2
  Minus3/1 -> Product6/2, Gain4/1
  Minus4/1 -> Integrator1/1
  Product5/1 -> Minus5/1
  Minus1/1 -> Product5/1, Gain2/1
  Product3/1 -> Minus4/1
  Product6/1 -> Minus5/2
  Gain2/1 -> Minus2/1
  Minus2/1 -> Integrator/1
  E_beta_hat/1 -> Minus3/2

== system PMSM_Sensorless_ASMO_PLL/FOC//SVPWM Algorithm/Clark_Conv ==
  Ia : Inport
  Ib : Inport  Port=2
  Ic : Inport  Port=3
  Add : Sum  Inputs=+-  OutDataTypeStr=double
  Gain : Gain  Gain=sqrt(3)  ParamDataTypeStr=double
  Gain2 : Gain  Gain=0.5
  Gain3 : Gain  Gain=0.5
  Subtract : Sum  Inputs=+--  OutDataTypeStr=double
  Ialpha : Outport
  Ibeta : Outport  Port=2
  wires:
  Ia/1 -> Subtract/1
  Ib/1 -> Gain2/1
  Add/1 -> Gain/1
  Gain/1 -> Ibeta/1
  Ic/1 -> Gain3/1
  Gain2/1 -> Subtract/2, Add/1
  Gain3/1 -> Subtract/3, Add/2
  Subtract/1 -> Ialpha/1

== system PMSM_Sensorless_ASMO_PLL/FOC//SVPWM Algorithm/Clark_Conv1 ==
  Ia : Inport
  Ib : Inport  Port=2
  Ic : Inport  Port=3
  Add : Sum  Inputs=+-  OutDataTypeStr=double
  Gain : Gain  Gain=sqrt(3)  ParamDataTypeStr=double
  Gain2 : Gain  Gain=0.5
  Gain3 : Gain  Gain=0.5
  Subtract : Sum  Inputs=+--  OutDataTypeStr=double
  Ialpha : Outport
  Ibeta : Outport  Port=2
  wires:
  Subtract/1 -> Ialpha/1
  Gain3/1 -> Add/2, Subtract/3
  Gain2/1 -> Add/1, Subtract/2
  Ic/1 -> Gain3/1
  Gain/1 -> Ibeta/1
  Add/1 -> Gain/1
  Ib/1 -> Gain2/1
  Ia/1 -> Subtract/1

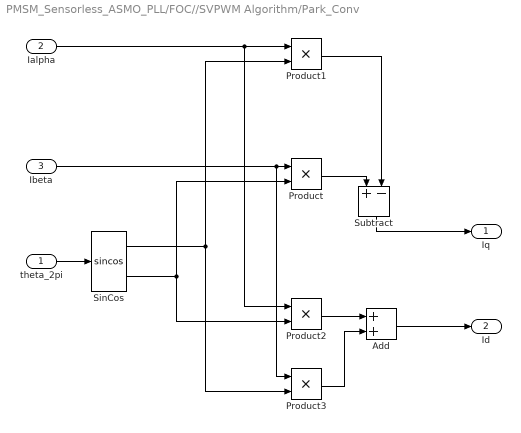
== system PMSM_Sensorless_ASMO_PLL/FOC//SVPWM Algorithm/Park_Conv ==
  theta_2pi : Inport
  Ialpha : Inport  Port=2
  Ibeta : Inport  Port=3
  Add : Sum
  Product{,1..3} (4 alike) : Product
  SinCos : Trigonometry  Operator=sincos
  Subtract : Sum  Inputs=+-
  Iq : Outport
  Id : Outport  Port=2
  wires:
  Ialpha/1 -> Product1/1, Product2/1
  Ibeta/1 -> Product3/1, Product/1
  theta_2pi/1 -> SinCos/1
  SinCos/2 -> Product2/2, Product/2
  SinCos/1 -> Product3/2, Product1/2
  Product1/1 -> Subtract/2
  Subtract/1 -> Iq/1
  Product/1 -> Subtract/1
  Product2/1 -> Add/1
  Product3/1 -> Add/2
  Add/1 -> Id/1

== system PMSM_Sensorless_ASMO_PLL/FOC//SVPWM Algorithm/Park_ReverseConv ==
  Uq : Inport
  Ud : Inport  Port=2
  theta_2pi : Inport  Port=3
  Add : Sum
  Product{,1..3} (4 alike) : Product
  SinCos : Trigonometry  Operator=sincos
  Subtract : Sum  Inputs=+-
  Ualpha : Outport
  Ubeta : Outport  Port=2
  wires:
  Uq/1 -> Product3/1, Product1/1
  Ud/1 -> Product2/1, Product/1
  SinCos/2 -> Product3/2, Product/2
  Product/1 -> Subtract/1
  SinCos/1 -> Product2/2, Product1/2
  Product1/1 -> Subtract/2
  Subtract/1 -> Ualpha/1
  Product2/1 -> Add/1
  Product3/1 -> Add/2
  Add/1 -> Ubeta/1
  theta_2pi/1 -> SinCos/1

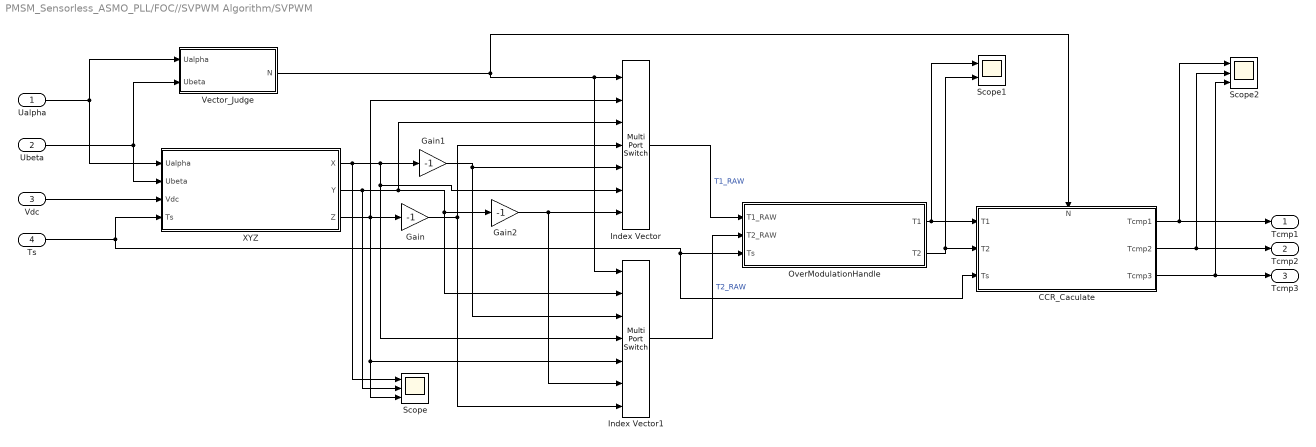
== system PMSM_Sensorless_ASMO_PLL/FOC//SVPWM Algorithm/SVPWM ==
  Ualpha : Inport
  Ubeta : Inport  Port=2
  Vdc : Inport  Port=3
  Ts : Inport  Port=4
  CCR_Caculate : Subsystem
      settings: PortSchema="{\"entries\":[{\"content\":{\"sides\":[{\"content\":{\"connectorIds\":[\"In1\",\"In2\",\"In3\"]},\"type\":\"ConnectorPlacement.EquallySpacedRectSide\",\"uuid\":\"41d89106-695f-4d7e-9c99-c52170b99868\"},{\"content\":{\"connectorIds\":[\"Out1\",\"Out2\",\"Out3\"],\"side\":\"RIGHT\"},\"type\":\"ConnectorPlacement.EquallySpacedRectSide\",\"uuid\":\"0fa1e6b9-7088-4c16-9dd3-c016449aae3e\"},{\"content\":{\"connectorIds\":[\"In4\"],\"side\":\"TOP\"},\"type\":\"ConnectorPlacement.EquallySpacedRectSide\",\"uuid\":\"6b702c00-29ab-49c7-a344-eb6fce3368af\"}]},\"type\":\"ConnectorPlacement.EquallySpacedConnector\",\"uuid\":\"c2f99839-550c-47c5-98fa-a115626cfb71\"}],\"packageUris\":[\"http://schema.mathworks.com/mf0/Connector/R2020b\"],\"version\":\"1.0\"}"
  Gain : Gain  Gain=-1
  Gain1 : Gain  Gain=-1
  Gain2 : Gain  Gain=-1
  Index Vector : MultiPortSwitch  Inputs=6  DiagnosticForDefault=None  SaturateOnIntegerOverflow=off  InputSameDT=off
  Index Vector1 : MultiPortSwitch  Inputs=6  DiagnosticForDefault=None  SaturateOnIntegerOverflow=off  InputSameDT=off
  OverModulationHandle : MATLAB Function  TreatAsAtomicUnit=on
  Scope : Scope  NumInputPorts=3
  Scope1 : Scope  NumInputPorts=2
  Scope2 : Scope  NumInputPorts=3
  Vector_Judge : Subsystem
  XYZ : Subsystem
  Tcmp1 : Outport
  Tcmp2 : Outport  Port=2
  Tcmp3 : Outport  Port=3
  wires:
  Ualpha/1 -> Vector_Judge/1(Ualpha), XYZ/1(Ualpha)
  Ubeta/1 -> Vector_Judge/2(Ubeta), XYZ/2(Ubeta)
  Vdc/1 -> XYZ/3(Vdc)
  Ts/1 -> CCR_Caculate/3(Ts), OverModulationHandle/3(Ts), XYZ/4(Ts)
  Vector_Judge/1(N) -> Index Vector1/1, Index Vector/1, CCR_Caculate/4(N)
  Index Vector1/1 -> OverModulationHandle/2(T2_RAW)  "T2_RAW"
  XYZ/3(Z) -> Scope/3, Index Vector1/5, Index Vector/2, Gain/1
  XYZ/2(Y) -> Scope/2, Index Vector1/2, Gain2/1, Index Vector/3
  Gain/1 -> Index Vector1/7, Index Vector/4
  XYZ/1(X) -> Scope/1, Index Vector1/4, Index Vector/6, Gain1/1
  Gain1/1 -> Index Vector1/3, Index Vector/5
  Gain2/1 -> Index Vector1/6, Index Vector/7
  Index Vector/1 -> OverModulationHandle/1(T1_RAW)  "T1_RAW"
  OverModulationHandle/1(T1) -> CCR_Caculate/1(T1), Scope1/1
  OverModulationHandle/2(T2) -> Scope1/2, CCR_Caculate/2(T2)
  CCR_Caculate/1(Tcmp1) -> Tcmp1/1, Scope2/1
  CCR_Caculate/2(Tcmp2) -> Tcmp2/1, Scope2/2
  CCR_Caculate/3(Tcmp3) -> Tcmp3/1, Scope2/3

== system PMSM_Sensorless_ASMO_PLL/Filter/LowpassFilter ==
  ln1 : Inport
  ln2 : Inport  Port=2
  ln3 : Inport  Port=3
  Lowpass filter1 : Subsystem
  Lowpass filter2 : Subsystem
  Lowpass filter3 : Subsystem
  a : Constant  Value=0.001
  Ia : Outport
  Ib : Outport  Port=2
  Ic : Outport  Port=3
  wires:
  ln2/1 -> Lowpass filter2/2(u(t))
  a/1 -> Lowpass filter3/1(K), Lowpass filter2/1(K), Lowpass filter1/1(K)
  ln1/1 -> Lowpass filter1/2(u(t))
  Lowpass filter1/1(Ia) -> Ia/1
  Lowpass filter2/1(Ib) -> Ib/1
  Lowpass filter3/1(Ic) -> Ic/1
  ln3/1 -> Lowpass filter3/2(u(t))

== system PMSM_Sensorless_ASMO_PLL/Filter/NoneFilter ==
  ln1 : Inport
  ln2 : Inport  Port=2
  ln3 : Inport  Port=3
  Ia : Outport
  Ib : Outport  Port=2
  Ic : Outport  Port=3
  wires:
  ln1/1 -> Ia/1
  ln2/1 -> Ib/1
  ln3/1 -> Ic/1

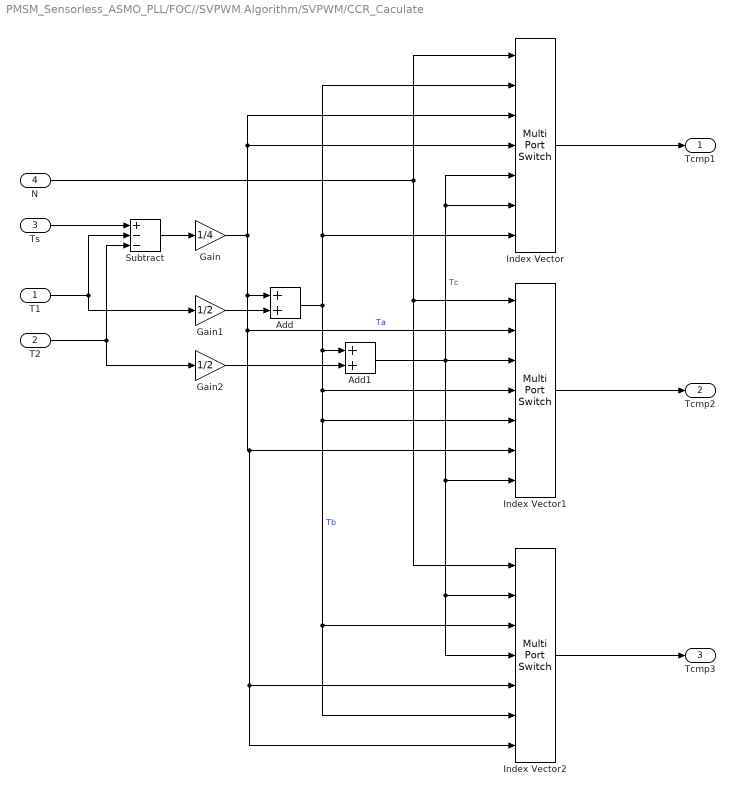
== system PMSM_Sensorless_ASMO_PLL/FOC//SVPWM Algorithm/SVPWM/CCR_Caculate ==
  T1 : Inport
  T2 : Inport  Port=2
  Ts : Inport  Port=3
  N : Inport  Port=4
  Add : Sum
  Add1 : Sum
  Gain : Gain  Gain=1/4
  Gain1 : Gain  Gain=1/2
  Gain2 : Gain  Gain=1/2
  Index Vector : MultiPortSwitch  Inputs=6  DiagnosticForDefault=None  SaturateOnIntegerOverflow=off  InputSameDT=off
  Index Vector1 : MultiPortSwitch  Inputs=6  DiagnosticForDefault=None  SaturateOnIntegerOverflow=off  InputSameDT=off
  Index Vector2 : MultiPortSwitch  Inputs=6  DiagnosticForDefault=None  SaturateOnIntegerOverflow=off  InputSameDT=off
  Subtract : Sum  Inputs=+--
  Tcmp1 : Outport
  Tcmp2 : Outport  Port=2
  Tcmp3 : Outport  Port=3
  wires:
  Ts/1 -> Subtract/1
  T1/1 -> Gain1/1, Subtract/2
  T2/1 -> Gain2/1, Subtract/3
  Subtract/1 -> Gain/1
  Gain/1 -> Index Vector2/7, Index Vector2/5, Index Vector1/6, Index Vector1/2, Add/1, Index Vector/4, Index Vector/3  "Ta"
  Gain1/1 -> Add/2
  Add/1 -> Index Vector1/5, Index Vector2/6, Index Vector2/3, Index Vector1/4, Add1/1, Index Vector/7, Index Vector/2  "Tb"
  Gain2/1 -> Add1/2
  Add1/1 -> Index Vector2/4, Index Vector2/2, Index Vector1/7, Index Vector1/3, Index Vector/6, Index Vector/5  "Tc"
  N/1 -> Index Vector2/1, Index Vector1/1, Index Vector/1
  Index Vector/1 -> Tcmp1/1
  Index Vector1/1 -> Tcmp2/1
  Index Vector2/1 -> Tcmp3/1

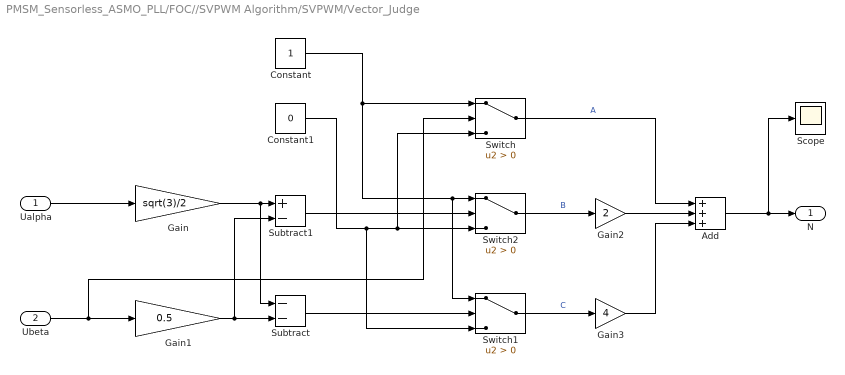
== system PMSM_Sensorless_ASMO_PLL/FOC//SVPWM Algorithm/SVPWM/Vector_Judge ==
  Ualpha : Inport
  Ubeta : Inport  Port=2
  Add : Sum  Inputs=+++
  Constant : Constant
  Constant1 : Constant  Value=0
  Gain : Gain  Gain=sqrt(3)/2
  Gain1 : Gain  Gain=0.5
  Gain2 : Gain  Gain=2
  Gain3 : Gain  Gain=4
  Scope : Scope
  Subtract : Sum  Inputs=--
  Subtract1 : Sum  Inputs=+-
  Switch : Switch  Criteria=u2 > Threshold  SaturateOnIntegerOverflow=off  InputSameDT=off
  Switch1 : Switch  Criteria=u2 > Threshold  SaturateOnIntegerOverflow=off  InputSameDT=off
  Switch2 : Switch  Criteria=u2 > Threshold  SaturateOnIntegerOverflow=off  InputSameDT=off
  N : Outport
  wires:
  Ualpha/1 -> Gain/1
  Ubeta/1 -> Gain1/1, Switch/2
  Switch/1 -> Add/1  "A"
  Switch1/1 -> Gain3/1  "C"
  Constant1/1 -> Switch2/3, Switch/3, Switch1/3
  Constant/1 -> Switch2/1, Switch1/1, Switch/1
  Switch2/1 -> Gain2/1  "B"
  Gain3/1 -> Add/3
  Add/1 -> Scope/1, N/1
  Gain2/1 -> Add/2
  Gain/1 -> Subtract/1, Subtract1/1
  Gain1/1 -> Subtract/2, Subtract1/2
  Subtract1/1 -> Switch2/2
  Subtract/1 -> Switch1/2

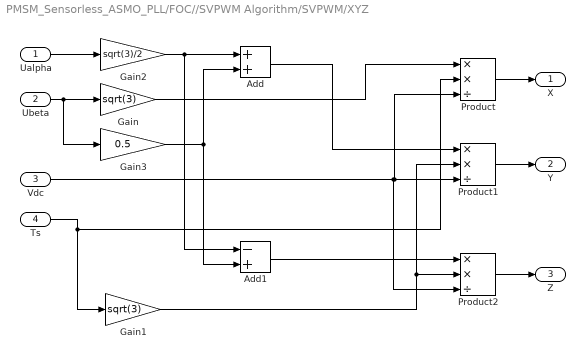
== system PMSM_Sensorless_ASMO_PLL/FOC//SVPWM Algorithm/SVPWM/XYZ ==
  Ualpha : Inport
  Ubeta : Inport  Port=2
  Vdc : Inport  Port=3
  Ts : Inport  Port=4
  Add : Sum
  Add1 : Sum  Inputs=-+
  Gain : Gain  Gain=sqrt(3)
  Gain1 : Gain  Gain=sqrt(3)
  Gain2 : Gain  Gain=sqrt(3)/2
  Gain3 : Gain  Gain=0.5
  Product : Product  Inputs=**/
  Product1 : Product  Inputs=**/
  Product2 : Product  Inputs=**/
  X : Outport
  Y : Outport  Port=2
  Z : Outport  Port=3
  wires:
  Ualpha/1 -> Gain2/1
  Gain/1 -> Product/1
  Ubeta/1 -> Gain3/1, Gain/1
  Ts/1 -> Product/2, Gain1/1
  Vdc/1 -> Product1/3, Product/3, Product2/3
  Product/1 -> X/1
  Gain2/1 -> Add1/1, Add/1
  Gain3/1 -> Add/2, Add1/2
  Add/1 -> Product1/1
  Gain1/1 -> Product2/2, Product1/2
  Product1/1 -> Y/1
  Add1/1 -> Product2/1
  Product2/1 -> Z/1

== system PMSM_Sensorless_ASMO_PLL/Filter/LowpassFilter/Lowpass filter1 ==
  K : Inport
  u(t) : Inport  Port=2
  Add : Sum
  Delay : Delay  DelayLength=1
  Product : Product
  Subtract : Sum  Inputs=+-
  Ia : Outport
  wires:
  Add/1 -> Ia/1, Delay/1
  Product/1 -> Add/1
  Subtract/1 -> Product/2
  Delay/1 -> Subtract/2, Add/2
  K/1 -> Product/1
  u(t)/1 -> Subtract/1

== system PMSM_Sensorless_ASMO_PLL/Filter/LowpassFilter/Lowpass filter2 ==
  K : Inport
  u(t) : Inport  Port=2
  Add : Sum
  Delay : Delay  DelayLength=1
  Product : Product
  Subtract : Sum  Inputs=+-
  Ib : Outport
  wires:
  u(t)/1 -> Subtract/1
  K/1 -> Product/1
  Delay/1 -> Add/2, Subtract/2
  Subtract/1 -> Product/2
  Product/1 -> Add/1
  Add/1 -> Delay/1, Ib/1

== system PMSM_Sensorless_ASMO_PLL/Filter/LowpassFilter/Lowpass filter3 ==
  K : Inport
  u(t) : Inport  Port=2
  Add : Sum
  Delay : Delay  DelayLength=1
  Product : Product
  Subtract : Sum  Inputs=+-
  Ic : Outport
  wires:
  Add/1 -> Ic/1, Delay/1
  Product/1 -> Add/1
  Subtract/1 -> Product/2
  Delay/1 -> Subtract/2, Add/2
  K/1 -> Product/1
  u(t)/1 -> Subtract/1

== matlab function PMSM_Sensorless_ASMO_PLL/MATLAB Function ==
  data: angle input; theta_2pi output
function theta_2pi = Angle_Conv(angle)

theta_2pi=mod(angle,2*pi);

== matlab function PMSM_Sensorless_ASMO_PLL/PLL1/MATLAB Function1 ==
  data: angle input; theta_2pi output
function theta_2pi = Angle_Conv(angle)

theta_2pi=mod(angle,2*pi);

== matlab function PMSM_Sensorless_ASMO_PLL/FOC//SVPWM Algorithm/CCR_Generator ==
  data: CNT input; Tcmp1 input; Tcmp2 input; Tcmp3 input; CH1 output; CH1N output; CH2 output; CH2N output; CH3 output; CH3N output
function[CH1,CH1N,CH2,CH2N,CH3,CH3N] = CCR_Generator(CNT,Tcmp1, Tcmp2, Tcmp3)

if (CNT<Tcmp1)
    CH1=0;
    CH1N=1;
else
    CH1=1;
    CH1N=0;
end
if (CNT<Tcmp2)
    CH2=0;
    CH2N=1;
else
    CH2=1;
    CH2N=0;
end
if (CNT<Tcmp3)
    CH3=0;
    CH3N=1;
else
    CH3=1;
    CH3N=0;
end
end

== matlab function PMSM_Sensorless_ASMO_PLL/FOC//SVPWM Algorithm/SVPWM/OverModulationHandle ==
  data: T1_RAW input; T2_RAW input; T1 output; T2 output; Ts input
function [T1,T2] = OverModulationHandle(T1_RAW, T2_RAW, Ts)
if((T1_RAW+T2_RAW)>Ts)
    T1=T1_RAW/(T1_RAW+T2_RAW)*Ts;
    T2=T2_RAW/(T1_RAW+T2_RAW)*Ts;
else
    T1=T1_RAW;
    T2=T2_RAW;
end
end

== matlab function PMSM_Sensorless_ASMO_PLL/PLL/MATLAB Function1 ==
  data: angle input; theta_2pi output
function theta_2pi = Angle_Conv(angle)

theta_2pi=mod(angle,2*pi);
